simulink model "Closedloop"  (R2015b)
settings: Solver=VariableStepAuto  StartTime=0.0  StopTime=300  FixedStep=DT  MaxStep=DT  RelTol=1e-3
values from neighbouring files (symbols this model uses):
  BT = 5    [Run_BorderTest.m]    (also in Run_FullProf.m = 20)
  Cp_opt = 0.4857    [Run_BorderTest.m]    (also in Run_FullProf.m)
  lambda_opt = 7.1    [Run_BorderTest.m]    (also in Run_FullProf.m)
  ng = 87.965    [Run_BorderTest.m]    (also in Run_FullProf.m)
  R = 35    [Run_BorderTest.m]    (also in Run_FullProf.m)
  Rho = 1.225    [Run_BorderTest.m]    (also in Run_FullProf.m)
undefined symbols (not defined in the file or in its folder): OutList, strmatch
libraries: simulink x1
settings Model: Creator=bjonkman  LastModifiedBy=alino
settings DataIOCC: SaveFormat=Array  SignalLoggingSaveFormat=ModelDataLogs  SaveOutput=off  SaveTime=off  SignalLoggingName=sigsOut
settings OptimizationCC: ExpressionDepthLimit=2147483647
settings DebuggingCC: SaveWithParameterizedLinksMsg=none  UnderspecifiedInitializationDetection=Classic  MergeDetectMultiDrivingBlocksExec=none  SignalResolutionControl=TryResolveAllWithWarning  MultiTaskDSMMsg=warning  MultiTaskCondExecSysMsg=none  FcnCallInpInsideContextMsg=EnableAllAsWarning  StateNameClashWarn=warning
settings HardwareCC: ProdBitPerPointer=32  ProdLargestAtomicFloat=None  ProdIntDivRoundTo=Undefined  ProdEndianess=Unspecified  ProdWordSize=32  ProdHWDeviceType=32-bit Generic  TargetUnknown=on
settings GRTTargetCC: GeneratePreprocessorConditionals=Disable all  CombineOutputUpdateFcns=off  GRTInterface=on
settings ConfigComp: CovModelRefEnable=Off

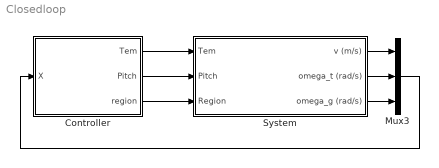
== system Closedloop ==
  Controller : Subsystem
  Mux3 : Mux  Inputs=3
  System : Subsystem
  wires:
  Mux3/1 -> Controller/1(X)
  Controller/1("Tem ") -> System/1(Tem)
  Controller/2(Pitch) -> System/2(Pitch)
  System/3(omega_g (rad/s)) -> Mux3/3
  System/2(omega_t (rad/s)) -> Mux3/2
  System/1(v (m/s)) -> Mux3/1
  Controller/3(region) -> System/3(Region)

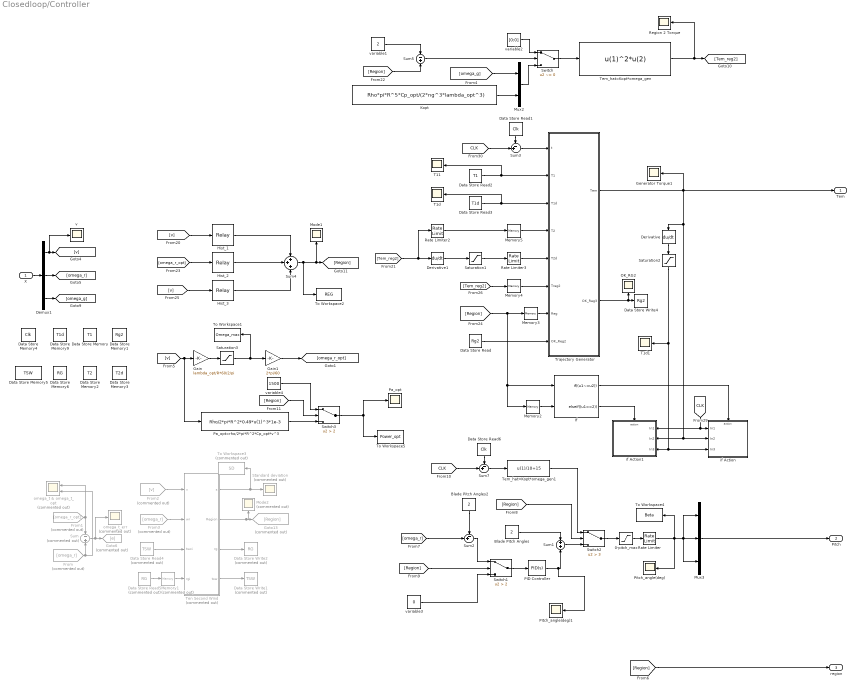
== system Closedloop/Controller ==
  X : Inport
  0-pitch_max : Saturate  UpperLimit=90  LowerLimit=2
  Blade Pitch Angles : Constant  Value=2
  Blade Pitch Angles2 : Constant  Value=2
  Data Store Memory : DataStoreMemory  DataStoreName=T1
  Data Store Memory1 : DataStoreMemory  DataStoreName=Rg2  InitialValue=1
  Data Store Memory2 : DataStoreMemory  DataStoreName=T2
  Data Store Memory3 : DataStoreMemory  DataStoreName=T2d
  Data Store Memory4 : DataStoreMemory  DataStoreName=Clk
  Data Store Memory5 : DataStoreMemory  DataStoreName=TSW  InitialValue=zeros(1,500)
  Data Store Memory6 : DataStoreMemory  DataStoreName=RG  InitialValue=[0 0 0]  OutDataTypeStr=double
  Data Store Memory9 : DataStoreMemory  DataStoreName=T1d
  Data Store Read : DataStoreRead  DataStoreName=Rg2  SampleTime=0
  Data Store Read1 : DataStoreRead  DataStoreName=Clk  SampleTime=0
  Data Store Read2 : DataStoreRead  DataStoreName=T1  SampleTime=0
  Data Store Read3 : DataStoreRead  DataStoreName=T1d  SampleTime=0
  Data Store Read4 : DataStoreRead  Commented=on  DataStoreName=TSW
  Data Store Read5 : DataStoreRead  Commented=on  DataStoreName=RG
  Data Store Read6 : DataStoreRead  DataStoreName=Clk  SampleTime=0
  Data Store Write1 : DataStoreWrite  Commented=on  DataStoreName=TSW
  Data Store Write2 : DataStoreWrite  Commented=on  DataStoreName=RG
  Data Store Write4 : DataStoreWrite  DataStoreName=Rg2
  Demux1 : Demux  Outputs=3
  Derivative : Derivative  CoefficientInTFapproximation=10
  Derivative1 : Derivative  CoefficientInTFapproximation=50
  From : From  Commented=on  GotoTag=omega_r
  From1 : From  Commented=on  GotoTag=omega_r_opt
  From2 : From  Commented=on  GotoTag=v
  From3 : From  Commented=on  GotoTag=omega_r
  Gain : Gain  Gain=lambda_opt/R*60/2/pi
  Gain1 : Gain  Gain=2*pi/60
  Generator Torque1 : Scope
  Goto13 : Goto  Commented=on  GotoTag=Region
  Goto6 : Goto  Commented=on  GotoTag=e
  Hist_1 : Relay  OnSwitchValue=3.3  OffSwitchValue=2.9  OnOutputValue=2  OffOutputValue=1
  Hist_2 : Relay  OnSwitchValue=2  OffSwitchValue=1.8
  Hist_3 : Relay  OnSwitchValue=24  OffSwitchValue=22  ZeroCross=off
  If : If  NumInputs=2  IfExpression=(u1~=u2)  ElseIfExpressions=(u1==2)  ShowElse=off
  "Kopt " : Constant  Value=Rho*pi*R^5*Cp_opt/(2*ng^3*lambda_opt^3)
  Memory1 : Memory  Commented=on
  Memory2 : Memory
  Memory3 : Memory  X0=2
  Memory4 : Memory
  Memory5 : Memory
  Mode1 : Scope
  Mode2 : Scope  Commented=on
  Mux2 : Mux  Inputs=2
  Mux3 : Mux  Inputs=3
  OK_RG2 : Scope
  PID Controller : simulink/Continuous/PID Controller  Controller=PID  TimeDomain=Continuous-time  SampleTime=-1  IntegratorMethod=Forward Euler  FilterMethod=Forward Euler  Form=Parallel  UseFilter=on  ControllerParametersSource=internal  P=100  I=30  D=1  N=100  InitialConditionSource=internal  InitialConditionForIntegrator=0  InitialConditionForFilter=0  ExternalReset=none  LimitOutput=off  UpperSaturationLimit=inf  LowerSaturationLimit=-inf  LinearizeAsGain=on  AntiWindupMode=none  Kb=1  TrackingMode=off  Kt=1  PParamMin=[]  PParamMax=[]  IParamMin=[]  IParamMax=[]  DParamMin=[]  DParamMax=[]  NParamMin=[]  NParamMax=[]  KbParamMin=[]  KbParamMax=[]  KtParamMin=[]  KtParamMax=[]  POutMin=[]  POutMax=[]  IOutMin=[]  IOutMax=[]  DOutMin=[]  DOutMax=[]  NOutMin=[]  NOutMax=[]  KbOutMin=[]  KbOutMax=[]  KtOutMin=[]  KtOutMax=[]  IntegratorOutMin=[]  IntegratorOutMax=[]  FilterOutMin=[]  FilterOutMax=[]  SumOutMin=[]  SumOutMax=[]  SumI1OutMin=[]  SumI1OutMax=[]  SumI2OutMin=[]  SumI2OutMax=[]  SumI3OutMin=[]  SumI3OutMax=[]  SumDOutMin=[]  SumDOutMax=[]  SaturationOutMin=[]  SaturationOutMax=[]  IntegratorContinuousStateAttributes=''  IntegratorStateMustResolveToSignalObject=off  IntegratorRTWStateStorageClass=Auto  FilterContinuousStateAttributes=''  FilterStateMustResolveToSignalObject=off  FilterRTWStateStorageClass=Auto  DifferentiatorICPrevScaledInput=0  DifferentiatorOutMin=[]  DifferentiatorOutMax=[]
  Pa_opt : Scope
  Pa_opt=rho/2*pi*R^2*Cp_opt*v^3 : Fcn  Expr=Rho/2*pi*R^2*0.49*u(1)^3*1e-3
  Pitch_angle(deg) : Scope
  Pitch_angle(deg)1 : Scope
  "Rate Limiter   " : RateLimiter  RisingSlewLimit=4  FallingSlewLimit=-4
  Rate Limiter2 : RateLimiter  RisingSlewLimit=50  FallingSlewLimit=-50
  Rate Limiter3 : RateLimiter  RisingSlewLimit=50  FallingSlewLimit=-50  SampleTimeMode=inherited
  Region 2 Torque : Scope
  Saturation1 : Saturate  UpperLimit=1000  LowerLimit=-1000  LinearizeAsGain=off  ZeroCross=off
  Saturation2 : Saturate  UpperLimit=500  LowerLimit=-500  ZeroCross=off
  Saturation3 : Saturate  UpperLimit=20.5  LowerLimit=0  ZeroCross=off
  Standard deviation : Scope  Commented=on
  Sum : Sum  Commented=on  Inputs=-+
  Sum1 : Sum  Inputs=+|+
  Sum2 : Sum  Inputs=-+|  SaturateOnIntegerOverflow=on
  Sum3 : Sum  Inputs=-+|
  Sum4 : Sum  Inputs=+++
  Sum5 : Sum  Inputs=-+
  Sum7 : Sum  Inputs=-+|
  Switch : Switch  Criteria=u2 ~= 0  Threshold=2
  Switch1 : Switch  Criteria=u2 > Threshold  Threshold=2  ZeroCross=off
  Switch2 : Switch  Criteria=u2 > Threshold  Threshold=3  ZeroCross=off
  Switch3 : Switch  Criteria=u2 > Threshold  Threshold=2  ZeroCross=off
  T11 : Scope
  T1d : Scope
  T1d1 : Scope
  Tem_hat=Kopt*omega_gen : Fcn  Expr=u(1)^2*u(2)
  Tem_hat=Kopt*omega_gen1 : Fcn  Expr=u(1)/10+15
  Ten Second Wind : MATLAB Function  Commented=on  TreatAsAtomicUnit=on
  To Workspace1 : ToWorkspace  VariableName=Omega_max  SaveFormat=Timeseries  SampleTime=-1
  To Workspace2 : ToWorkspace  VariableName=REG  SaveFormat=Timeseries  SampleTime=-1
  To Workspace3 : ToWorkspace  Commented=on  VariableName=SD  SaveFormat=Timeseries  SampleTime=-1
  To Workspace4 : ToWorkspace  VariableName=Beta  SaveFormat=Timeseries  SampleTime=-1
  To Workspace5 : ToWorkspace  VariableName=Power_opt  SaveFormat=Timeseries  SampleTime=-1
  Trajectory Generator : MATLAB Function  TreatAsAtomicUnit=on
  if Action : Subsystem  TreatAsAtomicUnit=on
  if Action1 : Subsystem  TreatAsAtomicUnit=on
  omega_t & omega_t_opt : Scope  Commented=on  NumInputPorts=2
  omega_t_err : Scope  Commented=on
  v : Scope
  variable1 : Constant  Value=2
  variable2 : Constant  Value=[0;0]
  variable3 : Constant  Value=0
  variable4 : Constant  Value=1500
  "Tem " : Outport
  Pitch : Outport  Port=2
  region : Outport  Port=3
  wires:
  X/1 -> Demux1/1
  Demux1/1 -> v/1, [v]
  Demux1/2 -> [omega_r]
  Demux1/3 -> [omega_g]
  Sum/1 -> omega_t_err/1, Goto6/1
  From/1 -> Sum/2, omega_t & omega_t_opt/2
  From1/1 -> omega_t & omega_t_opt/1, Sum/1
  Tem_hat=Kopt*omega_gen/1 -> [Tem_reg2], Region 2 Torque/1
  Data Store Read3/1 -> T1d/1, Trajectory Generator/3(T1d)
  [Tem_reg2] -> Rate Limiter2/1, Derivative1/1
  [CLK] -> Sum3/2
  Data Store Read2/1 -> T11/1, Trajectory Generator/2(T1)
  Trajectory Generator/2(OK_Reg3) -> OK_RG2/1, Data Store Write4/1
  Data Store Read/1 -> Trajectory Generator/8(OK_Reg2)
  Memory2/1 -> If/2
  If/1 -> if Action/Action
  Derivative/1 -> Saturation2/1
  Sum3/1 -> Trajectory Generator/1(t)
  Data Store Read1/1 -> Sum3/1
  [CLK] -> if Action1/1(In1), if Action/1(In1)
  Derivative1/1 -> Saturation1/1
  Saturation1/1 -> Rate Limiter3/1
  Trajectory Generator/1(Tem) -> "Tem "/1, Generator Torque1/1, if Action/2(In2), if Action1/2(In2), Derivative/1
  Saturation2/1 -> if Action/3(In3), if Action1/3(In3), T1d1/1
  Hist_1/1 -> Sum4/1
  [omega_r_opt] -> Hist_2/1
  [v] -> Hist_1/1
  [v] -> Hist_3/1
  Hist_2/1 -> Sum4/2
  Hist_3/1 -> Sum4/3
  [Region] -> Sum5/2
  variable1/1 -> Sum5/1
  [Region] -> If/1, Memory2/1, Memory3/1
  Memory5/1 -> Trajectory Generator/4(T2)
  Rate Limiter3/1 -> Trajectory Generator/5(T2d)
  Rate Limiter2/1 -> Memory5/1
  [Tem_reg2] -> Memory4/1
  Memory4/1 -> Trajectory Generator/6(Treg2)
  If/2 -> if Action1/Action
  Sum5/1 -> Switch/2
  variable2/1 -> Switch/1
  Switch/1 -> Tem_hat=Kopt*omega_gen/1
  [omega_g] -> Mux2/1
  "Kopt "/1 -> Mux2/2
  Mux2/1 -> Switch/3
  From2/1 -> Ten Second Wind/1(v)
  Data Store Read4/1 -> Ten Second Wind/3(tswi)
  Ten Second Wind/1(s) -> To Workspace3/1, Standard deviation/1
  Ten Second Wind/2(Region) -> Mode2/1, Goto13/1
  Memory1/1 -> Ten Second Wind/4(rgi)
  Ten Second Wind/4(tsw) -> Data Store Write1/1
  Ten Second Wind/3(rg) -> Data Store Write2/1
  Data Store Read5/1 -> Memory1/1
  From3/1 -> Ten Second Wind/2(wr)
  [v] -> Pa_opt=rho/2*pi*R^2*Cp_opt*v^3/1, Gain/1
  Memory3/1 -> Trajectory Generator/7(Reg)
  [Region] -> region/1
  Blade Pitch Angles/1 -> Sum1/1
  PID Controller/1 -> Pitch_angle(deg)1/1, Sum1/2
  0-pitch_max/1 -> "Rate Limiter   "/1
  Sum1/1 -> Switch2/3
  "Rate Limiter   "/1 -> Mux3/3, Mux3/2, Mux3/1, To Workspace4/1, Pitch_angle(deg)/1
  Mux3/1 -> Pitch/1
  variable3/1 -> Switch1/3
  Sum2/1 -> Switch1/1
  Switch1/1 -> PID Controller/1
  [Region] -> Switch1/2
  Gain1/1 -> [omega_r_opt]
  Gain/1 -> Saturation3/1
  Saturation3/1 -> Gain1/1, To Workspace1/1
  Switch2/1 -> 0-pitch_max/1
  [Region] -> Switch2/2
  Tem_hat=Kopt*omega_gen1/1 -> Switch2/1
  Blade Pitch Angles2/1 -> Sum2/1
  [CLK] -> Sum7/2
  Sum7/1 -> Tem_hat=Kopt*omega_gen1/1
  Data Store Read6/1 -> Sum7/1
  [omega_r] -> Sum2/2
  Sum4/1 -> To Workspace2/1, [Region], Mode1/1
  Switch3/1 -> Pa_opt/1, To Workspace5/1
  Pa_opt=rho/2*pi*R^2*Cp_opt*v^3/1 -> Switch3/3
  [Region] -> Switch3/2
  variable4/1 -> Switch3/1

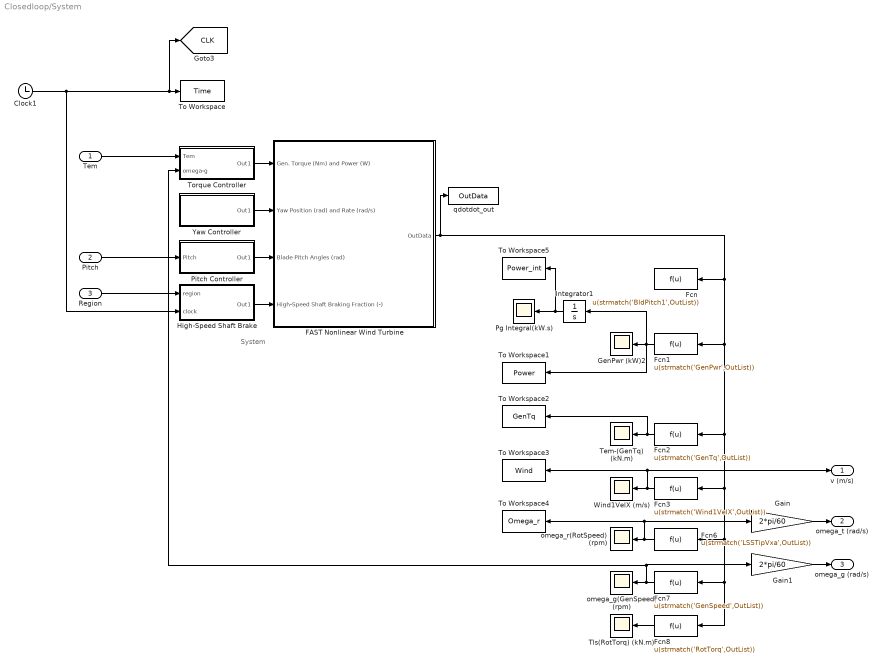
== system Closedloop/System ==
  note: System
  Tem : Inport
  Pitch : Inport  Port=2
  Region : Inport  Port=3
  Clock1 : Clock
  FAST Nonlinear Wind Turbine : Subsystem  mask(FAST Nonlinear Wind Turbine){}
      mask help: This block contains the FAST S-Function.
      mask init:
      | clear FAST_SFunc
  Fcn : Fcn  Expr=u(strmatch('BldPitch1',OutList))
  Fcn1 : Fcn  Expr=u(strmatch('GenPwr',OutList))
  Fcn2 : Fcn  Expr=u(strmatch('GenTq',OutList))
  Fcn3 : Fcn  Expr=u(strmatch('Wind1VelX',OutList))
  Fcn6 : Fcn  Expr=u(strmatch('LSSTipVxa',OutList))
  Fcn7 : Fcn  Expr=u(strmatch('GenSpeed',OutList))
  Fcn8 : Fcn  Expr=u(strmatch('RotTorq',OutList))
  Gain : Gain  Gain=2*pi/60
  Gain1 : Gain  Gain=2*pi/60
  GenPwr (kW)2 : Scope
  High-Speed Shaft Brake : Subsystem
  Integrator1 : Integrator
  Pg Integral(kW.s) : Scope
  Pitch Controller : Subsystem
  Tem-(GenTq) (kN.m) : Scope
  Tls(RotTorq) (kN.m) : Scope
  To Workspace : ToWorkspace  VariableName=Time  SampleTime=-1
  To Workspace1 : ToWorkspace  VariableName=Power  SaveFormat=Timeseries  SampleTime=-1
  To Workspace2 : ToWorkspace  VariableName=GenTq  SaveFormat=Timeseries  SampleTime=-1
  To Workspace3 : ToWorkspace  VariableName=Wind  SaveFormat=Timeseries  SampleTime=-1
  To Workspace4 : ToWorkspace  VariableName=Omega_r  SaveFormat=Timeseries  SampleTime=-1
  To Workspace5 : ToWorkspace  VariableName=Power_int  SaveFormat=Timeseries  SampleTime=-1
  Torque Controller : Subsystem
  Wind1VelX (m/s) : Scope
  Yaw Controller : Subsystem
  omega_g(GenSpeed) (rpm) : Scope
  omega_r(RotSpeed) (rpm) : Scope
  qdotdot_out : ToWorkspace  VariableName=OutData  SampleTime=-1
  v (m/s) : Outport
  omega_t (rad/s) : Outport  Port=2
  omega_g (rad/s) : Outport  Port=3
  tag scope: CLK=global
  wires:
  Clock1/1 -> [CLK], To Workspace/1, High-Speed Shaft Brake/2(clock)
  Torque Controller/1(Out1) -> FAST Nonlinear Wind Turbine/1(Gen. Torque (Nm) and Power (W))
  Yaw Controller/1(Out1) -> FAST Nonlinear Wind Turbine/2(Yaw Position (rad) and Rate (rad/s))
  Pitch Controller/1(Out1) -> FAST Nonlinear Wind Turbine/3(Blade Pitch Angles (rad))
  High-Speed Shaft Brake/1(Out1) -> FAST Nonlinear Wind Turbine/4(High-Speed Shaft Braking Fraction (-))
  Tem/1 -> Torque Controller/1(Tem)
  Pitch/1 -> Pitch Controller/1(Pitch)
  Fcn2/1 -> To Workspace2/1, Tem-(GenTq) (kN.m)/1
  Fcn3/1 -> To Workspace3/1, v (m/s)/1, Wind1VelX (m/s)/1
  Fcn6/1 -> To Workspace4/1, Gain/1, omega_r(RotSpeed) (rpm)/1
  Fcn7/1 -> Torque Controller/2(omega-g), Gain1/1, omega_g(GenSpeed) (rpm)/1
  Fcn8/1 -> Tls(RotTorq) (kN.m)/1
  FAST Nonlinear Wind Turbine/1(OutData) -> Fcn8/1, Fcn7/1, Fcn6/1, Fcn3/1, Fcn2/1, Fcn1/1, Fcn/1, qdotdot_out/1
  Gain/1 -> omega_t (rad/s)/1
  Gain1/1 -> omega_g (rad/s)/1
  Fcn1/1 -> Integrator1/1, To Workspace1/1, GenPwr (kW)2/1
  Integrator1/1 -> To Workspace5/1, Pg Integral(kW.s)/1
  Region/1 -> High-Speed Shaft Brake/1(region)

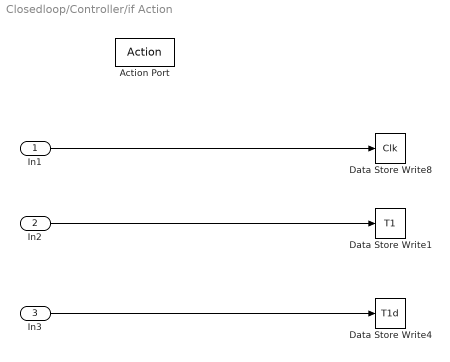
== system Closedloop/Controller/if Action ==
  In1 : Inport
  In2 : Inport  Port=2
  In3 : Inport  Port=3
  Action Port : ActionPort  ActionType=then
  Data Store Write1 : DataStoreWrite  DataStoreName=T1
  Data Store Write4 : DataStoreWrite  DataStoreName=T1d
  Data Store Write8 : DataStoreWrite  DataStoreName=Clk
  wires:
  In1/1 -> Data Store Write8/1
  In2/1 -> Data Store Write1/1
  In3/1 -> Data Store Write4/1

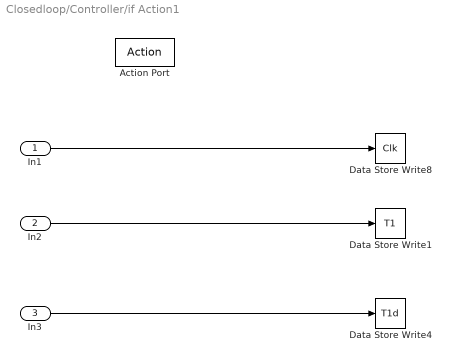
== system Closedloop/Controller/if Action1 ==
  In1 : Inport
  In2 : Inport  Port=2
  In3 : Inport  Port=3
  Action Port : ActionPort  ActionType=elseif
  Data Store Write1 : DataStoreWrite  DataStoreName=T1
  Data Store Write4 : DataStoreWrite  DataStoreName=T1d
  Data Store Write8 : DataStoreWrite  DataStoreName=Clk
  wires:
  In1/1 -> Data Store Write8/1
  In2/1 -> Data Store Write1/1
  In3/1 -> Data Store Write4/1

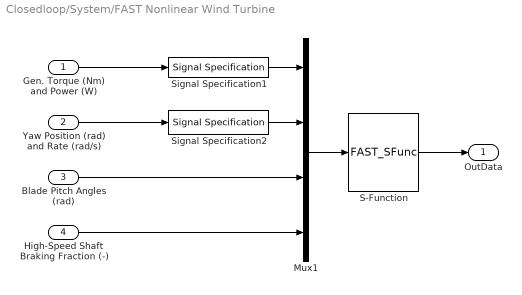
== system Closedloop/System/FAST Nonlinear Wind Turbine ==
  Gen. Torque (Nm) and Power (W) : Inport
  Yaw Position (rad) and Rate (rad/s) : Inport  Port=2
  Blade Pitch Angles (rad) : Inport  Port=3
  High-Speed Shaft Braking Fraction (-) : Inport  Port=4
  Mux1 : Mux
  S-Function : S-Function  FunctionName=FAST_SFunc  Parameters=FAST_InputFileName, TMax, 0  SFunctionDeploymentMode=off  EnableBusSupport=off
  Signal Specification1 : SignalSpecification  OutDataTypeStr=double  Dimensions=2
  Signal Specification2 : SignalSpecification  OutDataTypeStr=double  Dimensions=2
  OutData : Outport
  wires:
  Gen. Torque (Nm) and Power (W)/1 -> Signal Specification1/1
  S-Function/1 -> OutData/1
  Mux1/1 -> S-Function/1
  Blade Pitch Angles (rad)/1 -> Mux1/3
  Yaw Position (rad) and Rate (rad/s)/1 -> Signal Specification2/1
  Signal Specification1/1 -> Mux1/1
  Signal Specification2/1 -> Mux1/2
  High-Speed Shaft Braking Fraction (-)/1 -> Mux1/4

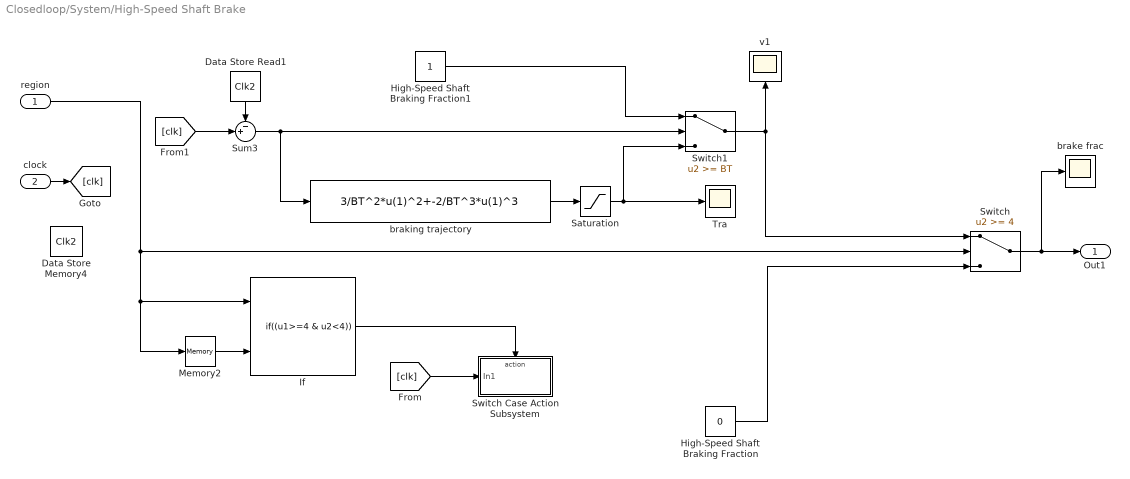
== system Closedloop/System/High-Speed Shaft Brake ==
  region : Inport
  clock : Inport  Port=2
  Data Store Memory4 : DataStoreMemory  DataStoreName=Clk2
  Data Store Read1 : DataStoreRead  DataStoreName=Clk2  SampleTime=0
  High-Speed Shaft Braking Fraction : Constant  Value=0
  High-Speed Shaft Braking Fraction1 : Constant
  If : If  NumInputs=2  IfExpression=(u1>=4 & u2<4)  ShowElse=off
  Memory2 : Memory
  Saturation : Saturate  UpperLimit=1  LowerLimit=0
  Sum3 : Sum  Inputs=-+|
  Switch : Switch  Threshold=4  ZeroCross=off
  Switch Case Action Subsystem : Subsystem  TreatAsAtomicUnit=on
  Switch1 : Switch  Threshold=BT  ZeroCross=off
  Tra : Scope
  brake frac : Scope
  braking trajectory : Fcn  Expr=3/BT^2*u(1)^2+-2/BT^3*u(1)^3
  v1 : Scope
  Out1 : Outport
  wires:
  Switch/1 -> brake frac/1, Out1/1
  High-Speed Shaft Braking Fraction/1 -> Switch/3
  Saturation/1 -> Switch1/3, Tra/1
  If/1 -> Switch Case Action Subsystem/Action
  [clk] -> Switch Case Action Subsystem/1(In1)
  [clk] -> Sum3/2
  Sum3/1 -> Switch1/2, braking trajectory/1
  Data Store Read1/1 -> Sum3/1
  braking trajectory/1 -> Saturation/1
  Memory2/1 -> If/2
  region/1 -> Switch/2, If/1, Memory2/1
  Switch1/1 -> v1/1, Switch/1
  High-Speed Shaft Braking Fraction1/1 -> Switch1/1
  clock/1 -> [clk]

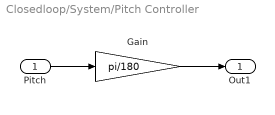
== system Closedloop/System/Pitch Controller ==
  Pitch : Inport
  Gain : Gain  Gain=pi/180
  Out1 : Outport
  wires:
  Pitch/1 -> Gain/1
  Gain/1 -> Out1/1

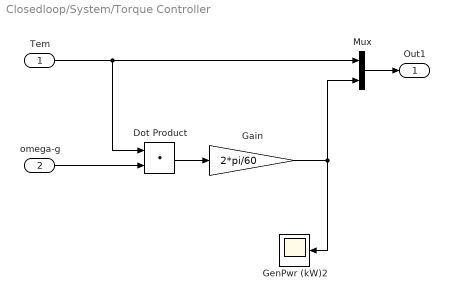
== system Closedloop/System/Torque Controller ==
  Tem : Inport
  omega-g : Inport  Port=2
  Dot Product : DotProduct  InputSameDT=on  OutDataTypeStr=Inherit: Inherit via internal rule
  Gain : Gain  Gain=2*pi/60
  GenPwr (kW)2 : Scope
  Mux : Mux  Inputs=2
  Out1 : Outport
  wires:
  Mux/1 -> Out1/1
  Tem/1 -> Dot Product/1, Mux/1
  omega-g/1 -> Dot Product/2
  Dot Product/1 -> Gain/1
  Gain/1 -> GenPwr (kW)2/1, Mux/2

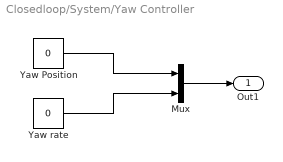
== system Closedloop/System/Yaw Controller ==
  Mux : Mux  Inputs=2
  Yaw Position : Constant  Value=0
  Yaw rate : Constant  Value=0
  Out1 : Outport
  wires:
  Mux/1 -> Out1/1
  Yaw Position/1 -> Mux/1
  Yaw rate/1 -> Mux/2

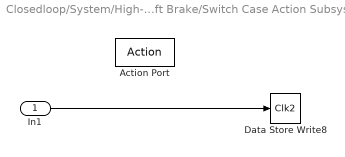
== system Closedloop/System/High-Speed Shaft Brake/Switch Case Action Subsystem ==
  In1 : Inport
  Action Port : ActionPort  ActionType=then
  Data Store Write8 : DataStoreWrite  DataStoreName=Clk2
  wires:
  In1/1 -> Data Store Write8/1

== matlab function Closedloop/Controller/Ten Second Wind ==
  data: v input; wr input; s output; tswi input; Region output; rg output; tsw output; rgi input
function [s,Region,rg,tsw] = fcn(v,wr,tswi,rgi)
    
    tsw=zeros(1,500);
    tsw(1:499)=tswi(2:500);
    tsw(500)=v;
    s=sqrt(var(tsw));
    rg=rgi;
    if v>25
        rg=[1;1;1];
    elseif v<(25-2*s)
        rg(3)=0;
    end
    if wr>(2)
        rg(2)=1;
    elseif wr<(2-2*s)
        rg(2)=0;
    end
    if v>(3+2*s)
        rg(1)=1;
    elseif v<3
        rg=[0;0;0];
    end
    
    Region=rg(1)+rg(2)+rg(3)+1;
end

== matlab function Closedloop/Controller/Trajectory Generator ==
  data: t input; Tem output; T1 input; T1d input; T2 input; T2d input; Treg2 input; Reg input; OK_Reg2 input; OK_Reg3 output
function [ Tem,OK_Reg3 ] = fcn1(t, T1, T1d, T2, T2d, Treg2, Reg, OK_Reg2)
if (Reg~=2)
    OK_Reg2=0;
    T=11;             %transition time
    T2=1.5e6/2/87.965;
    if (Reg~=3); T2=0; T=20; end
    T2d=0;            %desired T_dot
    if (t>T) 
        Tem=T2;
    else
        %T up trajectory(cubic spline)---------
        B1=T1;
        B2=T1d;
        B3=3*(T2-T1)/T^2-2*T1d/T-T2d/T;
        B4=2*(T1-T2)/T^3+T1d/T^2+T2d/T^2;

        thl=[B4 B3 B2 B1];
        Tem=polyval(thl,t); 
    end
elseif (OK_Reg2==0)
    T=7;
    if (abs(T1-Treg2)<1)
        OK_Reg2=1;
        Tem=Treg2;
    else
        %T down trajectory(cubic spline)---------
        B1=T1;
        B2=T1d;
        B3=3*(T2-T1)/T^2-2*T1d/T-T2d/T;
        B4=2*(T1-T2)/T^3+T1d/T^2+T2d/T^2;
        
        thl=[B4 B3 B2 B1];
        Tem=polyval(thl,t);
     end
else
    Tem=Treg2;
end
OK_Reg3=OK_Reg2;
end
